simulink library "ad_mem_any"  (R2017a)
settings: Solver=VariableStepAuto  StartTime=0.0  StopTime=10.0  RelTol=1e-3
libraries: ad_mem_base x2, ad_mem_any x2
settings Model: Creator=eruffaldi  LastModifiedBy=eruffaldi

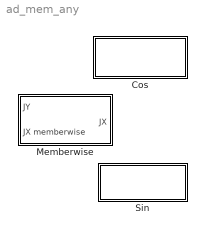
== system ad_mem_any ==
  Cos : Subsystem
      mask Display: disp('cos(x)');
  Memberwise : Subsystem
  Sin : Subsystem
      mask Display: disp('sin(x)');

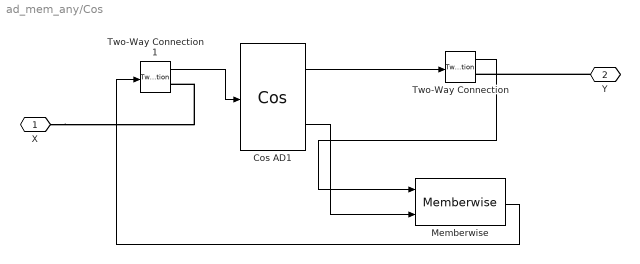
== system ad_mem_any/Cos ==
  Cos AD1 : ad_mem_base/Cos  SystemSampleTime=-1
      settings: SourceProductName=AutoDiff
  Memberwise : ad_mem_any/Memberwise
  Two-Way Connection : TwoWayConnection
  Two-Way Connection1 : TwoWayConnection
  X : PMIOPort  Port=1  Side=Left
  Y : PMIOPort  Port=2  Side=Right
  wires:
  Two-Way Connection1/1 -> Cos AD1/1
  Cos AD1/1 -> Two-Way Connection/1
  Cos AD1/2 -> Memberwise/2
  Two-Way Connection/1 -> Memberwise/1
  Memberwise/1 -> Two-Way Connection1/1
  connections:
  Y/RConn1 -- Two-Way Connection/RConn1
  X/RConn1 -- Two-Way Connection1/RConn1

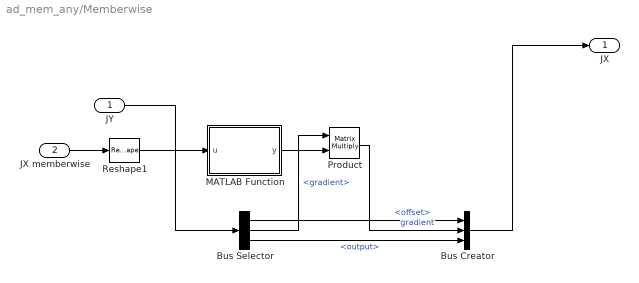
== system ad_mem_any/Memberwise ==
  JY : Inport
  JX memberwise : Inport  Port=2
  Bus Creator : BusCreator  Inputs='offset','gradient','output'
  Bus Selector : BusSelector  OutputSignals=offset,gradient,output
  MATLAB Function : MATLAB Function  TreatAsAtomicUnit=on
  Product : Product  Multiplication=Matrix(*)
  Reshape1 : Reshape  OutputDimensionality=Column vector (2-D)
  JX : Outport
  wires:
  JY/1 -> Bus Selector/1
  Reshape1/1 -> MATLAB Function/1(u)
  MATLAB Function/1(y) -> Product/2
  JX memberwise/1 -> Reshape1/1
  Bus Selector/2 -> Product/1  "<gradient>"
  Bus Selector/1 -> Bus Creator/1  "<offset>"
  Product/1 -> Bus Creator/2  "gradient"
  Bus Selector/3 -> Bus Creator/3  "<output>"
  Bus Creator/1 -> JX/1

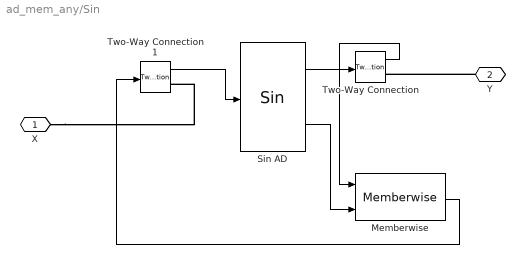
== system ad_mem_any/Sin ==
  Memberwise : ad_mem_any/Memberwise
  Sin AD : ad_mem_base/Sin
      settings: SourceProductName=AutoDiff
  Two-Way Connection : TwoWayConnection
  Two-Way Connection1 : TwoWayConnection
  X : PMIOPort  Port=1  Side=Left
  Y : PMIOPort  Port=2  Side=Right
  wires:
  Sin AD/1 -> Two-Way Connection/1
  Two-Way Connection1/1 -> Sin AD/1
  Sin AD/2 -> Memberwise/2
  Memberwise/1 -> Two-Way Connection1/1
  Two-Way Connection/1 -> Memberwise/1
  connections:
  X/RConn1 -- Two-Way Connection1/RConn1
  Y/RConn1 -- Two-Way Connection/RConn1

== matlab function ad_mem_any/Memberwise/MATLAB Function ==
  data: u input; y output
function y = fcn(u)

y = diag(u);
